simulink model "motor_dc_simulink"  (R2026a)
settings: Solver=ode45  StopTime=2
settings Model: Creator=ghass  LastModifiedBy=ghass

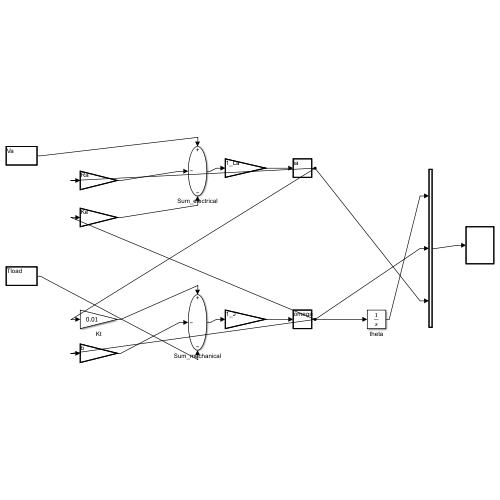
[thumbnail: Simulink's stored preview of the top-level diagram]
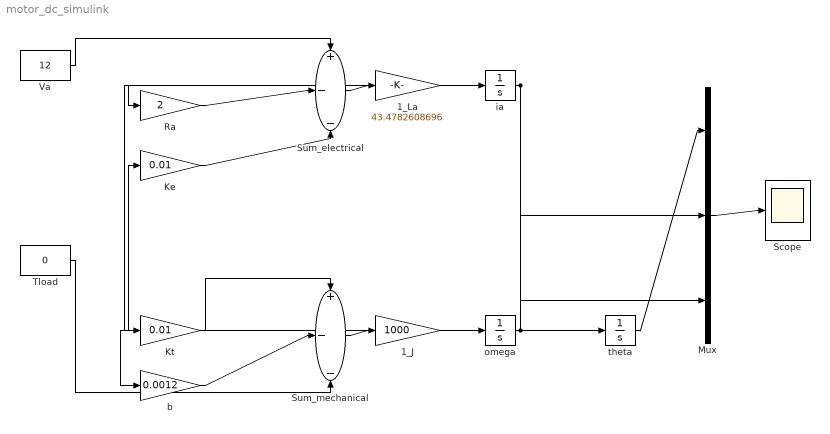
== system motor_dc_simulink ==
  1_J : Gain  Gain=1000
  1_La : Gain  Gain=43.4782608696
  Ke : Gain  Gain=0.01
  Kt : Gain  Gain=0.01
  Mux : Mux  Inputs=3
  Ra : Gain  Gain=2
  Scope : Scope
  Sum_electrical : Sum  Inputs=+--
  Sum_mechanical : Sum  Inputs=+--
  Tload : Constant  Value=0
  Va : Constant  Value=12
  b : Gain  Gain=0.0012
  ia : Integrator
  omega : Integrator
  theta : Integrator
  wires:
  Va/1 -> Sum_electrical/1
  ia/1 -> Ra/1, Kt/1, Mux/3
  Ra/1 -> Sum_electrical/2
  omega/1 -> Ke/1, b/1, theta/1, Mux/2
  Ke/1 -> Sum_electrical/3
  Sum_electrical/1 -> 1_La/1
  1_La/1 -> ia/1
  Kt/1 -> Sum_mechanical/1
  b/1 -> Sum_mechanical/2
  Tload/1 -> Sum_mechanical/3
  Sum_mechanical/1 -> 1_J/1
  1_J/1 -> omega/1
  theta/1 -> Mux/1
  Mux/1 -> Scope/1
